simulink model "mixer_old"  (R2024b)
settings: Solver=FixedStepAuto  StartTime=0.0  StopTime=10.0  RelTol=1e-3
undefined symbols (not defined in the file or in its folder): MC_AIRMODE, MOT_SLEW_MAX, THR_MDL_FAC
libraries: simulink x58
(part 1 of 3)
settings Model: DataDictionary=nextpilot_datadict.sldd  Creator=DELL  LastModifiedBy=CETCA
settings DebuggingCC: UnconnectedInputMsg=warning  UnconnectedOutputMsg=warning  UnconnectedLineMsg=warning
settings ModelReferenceCC: EnableRefExpFcnMdlSchedulingChecks=on
settings RTWCC: GPUComputeCapability=3.5  DLArmComputeVersion=19.05

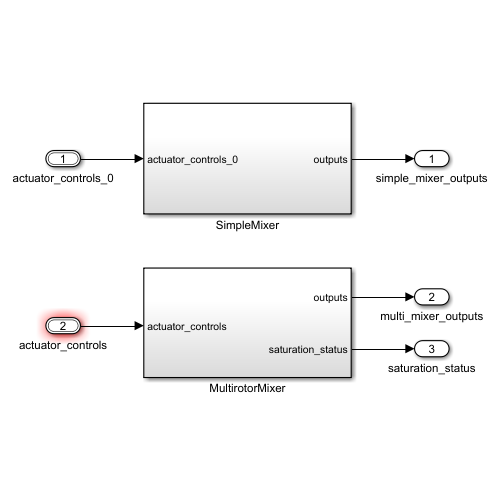
[thumbnail: Simulink's stored preview of the top-level diagram]
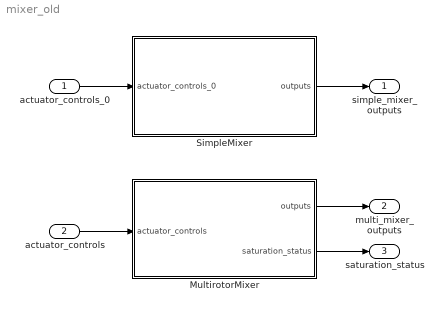
== system mixer_old ==
  actuator_controls_0 : Inport  OutDataTypeStr=Bus: actuator_controls_s
  actuator_controls : Inport  Port=2  OutDataTypeStr=Bus: px4_actuator_controls
  MultirotorMixer : Subsystem
  SimpleMixer : Subsystem
  simple_mixer_outputs : Outport
  multi_mixer_outputs : Outport  Port=2
  saturation_status : Outport  Port=3
  wires:
  actuator_controls/1 -> MultirotorMixer/1(actuator_controls)
  SimpleMixer/1(outputs) -> simple_mixer_outputs/1
  MultirotorMixer/1(outputs) -> multi_mixer_outputs/1
  MultirotorMixer/2(saturation_status) -> saturation_status/1
  actuator_controls_0/1 -> SimpleMixer/1(actuator_controls_0)

== system mixer_old/MultirotorMixer ==
  Bus Element In : Inport  PortName=actuator_controls  Element=control
  Bus Selector : BusSelector  OutputSignals=motor_neg,motor_pos,outputs
  Constant : Constant  Value=MC_AIRMODE
  Merge : Merge  Inputs=3
  Mux : Mux  Inputs=2
  Saturation : Saturate  UpperLimit=1.0  LowerLimit=-1.0
      settings: AttributesFormatString=[%<LowerLimit>, %<UpperLimit>]
  Saturation1 : Saturate  UpperLimit=1.0  LowerLimit=0.0
      settings: AttributesFormatString=[%<LowerLimit>, %<UpperLimit>]
  Selector : Selector  InputPortWidth=8  IndexOptions=Index vector (dialog)  Indices=[1 2 3]  OutputSizes=1
  Selector1 : Selector  InputPortWidth=8  IndexOptions=Index vector (dialog)  Indices=4  OutputSizes=1
  Switch Case : SwitchCase  CaseConditions={1 2}
  apply_thrust_model : Subsystem
  config_quad_x : Constant  Value=[-0.707107, 0.707107, 1.000000, 1.000000; 0.707107, -0.707107, 1.000000, 1.000000; 0.707107, 0.707107, -1.000000, 1.000000; -0.707107, -0.707107, -1.000000, 1.000000]  OutDataTypeStr=single
  mix_airmode_disabled : Subsystem
  mix_airmode_rp : Subsystem
  mix_airmode_rpy : Subsystem
  update_saturation_status : Subsystem
  outputs : Outport
  saturation_status : Outport  Port=2
  wires:
  Bus Element In/1 -> Selector1/1, Selector/1
  Selector/1 -> Saturation/1
  Selector1/1 -> Saturation1/1
  Saturation/1 -> Mux/1  "roll pitch yaw"
  Saturation1/1 -> Mux/2  "thrust"
  mix_airmode_rp/1(out) -> Merge/1
  mix_airmode_disabled/1(out) -> Merge/3
  Constant/1 -> Switch Case/1
  Switch Case/1 -> mix_airmode_rp/Action
  Switch Case/2 -> mix_airmode_rpy/Action
  Switch Case/3 -> mix_airmode_disabled/Action
  Mux/1 -> [four_channel]
  Merge/1 -> Bus Selector/1
  Bus Selector/1 -> [motor_neg]  "<motor_neg>"
  Bus Selector/2 -> [motor_pos]  "<motor_pos>"
  Bus Selector/3 -> apply_thrust_model/1(input)  "<outputs>"
  [motor_neg] -> update_saturation_status/2(motor_neg)
  [motor_pos] -> update_saturation_status/3(motor_pos)
  apply_thrust_model/2(clipping) -> update_saturation_status/1(clipping)
  apply_thrust_model/1(outputs) -> outputs/1
  update_saturation_status/1(saturation_status) -> saturation_status/1
  config_quad_x/1 -> [scale]
  [four_channel] -> mix_airmode_rp/1(four_input)
  [scale] -> mix_airmode_rp/2(scale)
  [four_channel] -> mix_airmode_rpy/1(four_input1)
  [scale] -> mix_airmode_rpy/2(scale1)
  mix_airmode_rpy/1(out1) -> Merge/2
  [four_channel] -> mix_airmode_disabled/1(four_input)
  [scale] -> mix_airmode_disabled/2(scale)
  [scale] -> update_saturation_status/4(scales)

== system mixer_old/SimpleMixer ==
  Bus Element In{,1..4} (5 alike) : Inport  PortName=actuator_controls_0  Element=control
  Constant{,1..19} (20 alike) : Constant  Value=[1 1]  OutDataTypeStr=single
  Constant{20..24} (5 alike) : Constant  OutDataTypeStr=single
  Mux : Mux  Inputs=5
  Selector : Selector  InputPortWidth=8  IndexOptions=Index vector (dialog)  Indices=[1 7]  OutputSizes=1
  Selector1 : Selector  InputPortWidth=8  IndexOptions=Index vector (dialog)  Indices=[1 7]  OutputSizes=1
  Selector2 : Selector  InputPortWidth=8  IndexOptions=Index vector (dialog)  Indices=[3 2]  OutputSizes=1
  Selector3 : Selector  InputPortWidth=8  IndexOptions=Index vector (dialog)  Indices=[3 2]  OutputSizes=1
  Selector4 : Selector  InputPortWidth=8  IndexOptions=Index vector (dialog)  Indices=4  OutputSizes=1
  Sum of Elements{,1..3} (4 alike) : Sum  Inputs=+
  scale : Subsystem
  scale1 : Subsystem
  scale2 : Subsystem
  scale3 : Subsystem
  scale4 : Subsystem
  outputs : Outport
  wires:
  Sum of Elements/1 -> [aileron_left]
  Sum of Elements1/1 -> [aileron_right]
  Sum of Elements3/1 -> [v_right]
  Sum of Elements2/1 -> [v_left]
  scale4/1(output) -> [prop]
  Bus Element In/1 -> Selector/1
  Bus Element In1/1 -> Selector1/1
  Bus Element In2/1 -> Selector2/1
  Bus Element In3/1 -> Selector3/1
  Bus Element In4/1 -> Selector4/1
  Constant4/1 -> scale/6(max)
  Selector/1 -> scale/1(input)
  Constant/1 -> scale/2(negative_scale)
  Constant3/1 -> scale/5(min)
  Constant1/1 -> scale/3(positive_scale)
  Constant2/1 -> scale/4(offset)
  scale/1(output) -> Sum of Elements/1
  scale1/1(output) -> Sum of Elements1/1
  Selector1/1 -> scale1/1(input)
  Constant5/1 -> scale1/2(negative_scale)
  Constant6/1 -> scale1/3(positive_scale)
  Constant7/1 -> scale1/4(offset)
  Constant8/1 -> scale1/5(min)
  Constant9/1 -> scale1/6(max)
  scale2/1(output) -> Sum of Elements2/1
  Selector2/1 -> scale2/1(input)
  Selector3/1 -> scale3/1(input)
  scale3/1(output) -> Sum of Elements3/1
  Selector4/1 -> scale4/1(input)
  Constant20/1 -> scale4/2(negative_scale)
  Constant10/1 -> scale2/2(negative_scale)
  Constant11/1 -> scale2/3(positive_scale)
  Constant12/1 -> scale2/4(offset)
  Constant13/1 -> scale2/5(min)
  Constant14/1 -> scale2/6(max)
  Constant15/1 -> scale3/2(negative_scale)
  Constant16/1 -> scale3/3(positive_scale)
  Constant17/1 -> scale3/4(offset)
  Constant18/1 -> scale3/5(min)
  Constant19/1 -> scale3/6(max)
  Constant21/1 -> scale4/3(positive_scale)
  Constant22/1 -> scale4/4(offset)
  Constant23/1 -> scale4/5(min)
  Constant24/1 -> scale4/6(max)
  [v_left] -> Mux/3
  [aileron_right] -> Mux/2
  [v_right] -> Mux/4
  [aileron_left] -> Mux/1
  [prop] -> Mux/5
  Mux/1 -> outputs/1

== system mixer_old/MultirotorMixer/apply_thrust_model ==
  input : Inport
  slew_rate_limit : Subsystem
  thrust_model : Subsystem
  outputs : Outport
  clipping : Outport  Port=2
  wires:
  input/1 -> thrust_model/1(input)
  thrust_model/1(outputs) -> slew_rate_limit/1(input)
  slew_rate_limit/2(clipping) -> clipping/1
  slew_rate_limit/1(output1) -> outputs/1

== system mixer_old/MultirotorMixer/mix_airmode_disabled ==
  four_input : Inport
  scale : Inport  Port=2
  Action Port : ActionPort  ActionPortLabel=default:
  Bus Selector3 : BusSelector  OutputSignals=outputs
  Bus Selector4 : BusSelector  OutputSignals=outputs
  Constant10 : Constant  OutDataTypeStr=single
  Constant11 : Constant  OutDataTypeStr=single
  Constant12 : Constant  Value=0  OutDataTypeStr=single
  Constant13 : Constant  OutDataTypeStr=single
  Constant14 : Constant  Value=0  OutDataTypeStr=single
  Constant9 : Constant  Value=0  OutDataTypeStr=single
  four_input1 : InportShadow
  minimize_saturation : Subsystem
  minimize_saturation1 : Subsystem
  minimize_saturation2 : Subsystem
  mix_yaw : Subsystem
  reduce_only : Constant  Value=0  OutDataTypeStr=single
  reduce_only1 : Constant  Value=0  OutDataTypeStr=single
  reduce_only2 : Constant  Value=0  OutDataTypeStr=single
  scale1 : InportShadow  Port=2
  scale2 : InportShadow  Port=2
  scale3 : InportShadow  Port=2
  out : Outport
  wires:
  scale/1 -> minimize_saturation/2(scale)
  reduce_only/1 -> minimize_saturation/5(reduce_only)
  Constant9/1 -> minimize_saturation/3(min_out)
  four_input/1 -> minimize_saturation/1(inputs)
  Constant10/1 -> minimize_saturation/4(max_out)
  Constant11/1 -> minimize_saturation1/4(max_out)
  Bus Selector3/1 -> minimize_saturation1/1(inputs)  "<outputs>"
  Constant12/1 -> minimize_saturation1/3(min_out)
  reduce_only1/1 -> minimize_saturation1/5(reduce_only)
  scale1/1 -> minimize_saturation1/2(scale)
  scale2/1 -> minimize_saturation2/2(scale)
  reduce_only2/1 -> minimize_saturation2/5(reduce_only)
  Constant14/1 -> minimize_saturation2/3(min_out)
  Bus Selector4/1 -> minimize_saturation2/1(inputs)  "<outputs>"
  Constant13/1 -> minimize_saturation2/4(max_out)
  minimize_saturation/1(out) -> Bus Selector3/1
  minimize_saturation1/1(out) -> Bus Selector4/1
  minimize_saturation2/1(out) -> mix_yaw/1(inputs)
  four_input1/1 -> mix_yaw/2(four_input)
  scale3/1 -> mix_yaw/3(scale)
  mix_yaw/1(out) -> out/1

== system mixer_old/MultirotorMixer/mix_airmode_rp ==
  four_input : Inport
  scale : Inport  Port=2
  Action Port : ActionPort  ActionPortLabel=case [ 1 ]:
  Constant1 : Constant  Value=0  OutDataTypeStr=single
  Constant2 : Constant  OutDataTypeStr=single
  four_input1 : InportShadow
  minimize_saturation : Subsystem
  mix_without_yaw : Subsystem
  mix_yaw : Subsystem
  reduce_only : Constant  Value=0  OutDataTypeStr=single
  scale1 : InportShadow  Port=2
  scale2 : InportShadow  Port=2
  out : Outport
  wires:
  reduce_only/1 -> minimize_saturation/5(reduce_only)
  four_input1/1 -> mix_yaw/2(four_input)
  Constant1/1 -> minimize_saturation/3(min_out)
  Constant2/1 -> minimize_saturation/4(max_out)
  minimize_saturation/1(out) -> mix_yaw/1(inputs)
  mix_yaw/1(out) -> out/1
  four_input/1 -> mix_without_yaw/1(four_input)
  scale/1 -> mix_without_yaw/2(scale)
  scale1/1 -> minimize_saturation/2(scale)
  mix_without_yaw/1(outputs) -> minimize_saturation/1(inputs)
  scale2/1 -> mix_yaw/3(scale)

== system mixer_old/MultirotorMixer/mix_airmode_rpy ==
  four_input1 : Inport
  scale1 : Inport  Port=2
  Action Port : ActionPort  ActionPortLabel=case [ 2 ]:
  Bus Selector : BusSelector  OutputSignals=outputs
  Constant6 : Constant  Value=0  OutDataTypeStr=single
  Constant7 : Constant  OutDataTypeStr=single
  Constant8 : Constant  Value=0  OutDataTypeStr=single
  Constant9 : Constant  OutDataTypeStr=single
  full_mixing : Subsystem
  minimize_saturation : Subsystem
  minimize_saturation1 : Subsystem
  reduce_only : Constant  Value=0  OutDataTypeStr=single
  reduce_only1 : Constant  Value=0  OutDataTypeStr=single
  scale2 : InportShadow  Port=2
  scale3 : InportShadow  Port=2
  out1 : Outport
  wires:
  four_input1/1 -> full_mixing/1(four_input)
  scale1/1 -> full_mixing/2(scale)
  scale2/1 -> minimize_saturation/2(scale)
  reduce_only/1 -> minimize_saturation/5(reduce_only)
  Constant6/1 -> minimize_saturation/3(min_out)
  full_mixing/1(outputs) -> minimize_saturation/1(inputs)
  Constant7/1 -> minimize_saturation/4(max_out)
  scale3/1 -> minimize_saturation1/2(scale)
  Constant8/1 -> minimize_saturation1/3(min_out)
  Constant9/1 -> minimize_saturation1/4(max_out)
  reduce_only1/1 -> minimize_saturation1/5(reduce_only)
  minimize_saturation1/1(out) -> out1/1
  minimize_saturation/1(out) -> Bus Selector/1
  Bus Selector/1 -> minimize_saturation1/1(inputs)  "<outputs>"

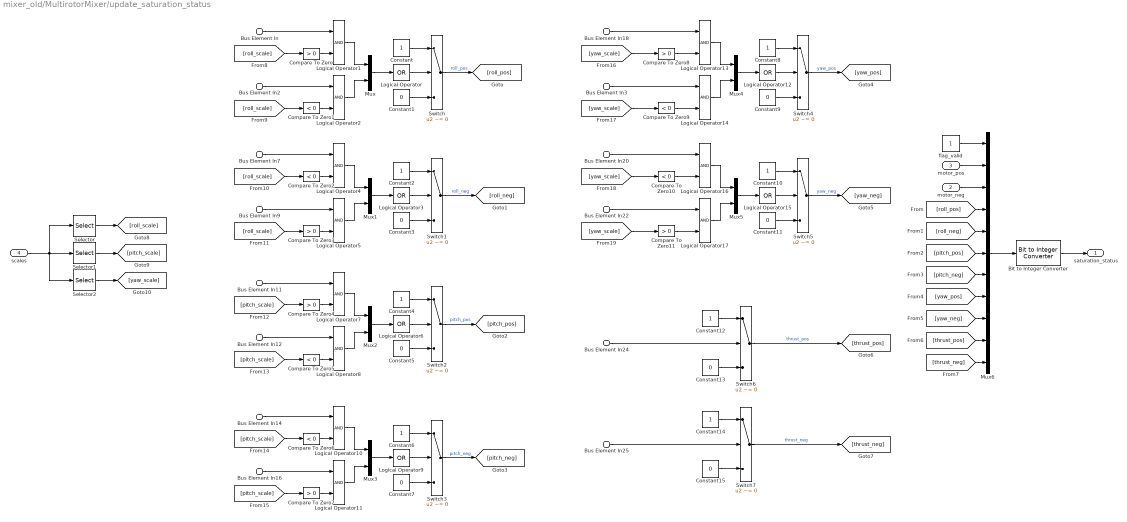
== system mixer_old/MultirotorMixer/update_saturation_status ==
  Bus Element In{,7,11,14,18,20,24} (7 alike) : Inport  PortName=clipping  Element=clipping_high
  Bus Element In{2,9,12,16,25} (5 alike) : Inport  PortName=clipping  Element=clipping_low_roll_pitch
  Bus Element In3 : Inport  PortName=clipping  Element=clipping_low_yaw
  Bus Element In22 : Inport  PortName=clipping  Element=clipping_low_yaw
  motor_neg : Inport  Port=2
  motor_pos : Inport  Port=3
  scales : Inport  Port=4
  Bit to Integer Converter : simulink/Logic and Bit Operations/Bit to Integer Converter  nbits=11  bitOrder=MSB first  signedOutputValues=Unsigned  outDtype=Inherit via internal rule  outDtypeSigned=Inherit via internal rule
      settings: LibrarySourceBlock=|
      | commutil2/Bit to Integer
      | Converter
  Compare To Zero{,3..4,7..8,11} (6 alike) : simulink/Logic and Bit Operations/Compare To Zero  relop=>  OutDataTypeStr=boolean
  Compare To Zero{1..2,5..6,9..10} (6 alike) : simulink/Logic and Bit Operations/Compare To Zero  relop=<  OutDataTypeStr=boolean
  Constant{,2,4,6,8,10,12,14} (8 alike) : Constant  OutDataTypeStr=single
  Constant{1,3,5,7,9,11,13,15} (8 alike) : Constant  Value=0  OutDataTypeStr=single
  Logical Operator{,3,6,9,12,15} (6 alike) : Logic  Operator=OR  Inputs=1  AllPortsSameDT=off  OutDataTypeStr=boolean
  Logical Operator{1..2,4..5,7..8,10..11,13..14,16..17} (12 alike) : Logic  AllPortsSameDT=off  OutDataTypeStr=boolean
  Mux{,1..5} (6 alike) : Mux  Inputs=2
  Mux6 : Mux  Inputs=11
  Selector : Selector  NumberOfDimensions=2  InputPortWidth=3  IndexOptions=Select all,Index vector (dialog)  Indices=[1 3],1  OutputSizes=1,1
  Selector1 : Selector  NumberOfDimensions=2  InputPortWidth=3  IndexOptions=Select all,Index vector (dialog)  Indices=[1 3],2  OutputSizes=1,1
  Selector2 : Selector  NumberOfDimensions=2  InputPortWidth=3  IndexOptions=Select all,Index vector (dialog)  Indices=[1 3],3  OutputSizes=1,1
  Switch{,1..7} (8 alike) : Switch  Criteria=u2 ~= 0  SaturateOnIntegerOverflow=off  InputSameDT=off
  flag_valid : Constant  OutDataTypeStr=single
  saturation_status : Outport
  wires:
  Switch/1 -> [roll_pos]  "roll_pos"
  Constant/1 -> Switch/1
  Constant1/1 -> Switch/3
  Logical Operator/1 -> Switch/2
  Bus Element In/1 -> Logical Operator1/1
  Compare To Zero/1 -> Logical Operator1/2
  [roll_scale] -> Compare To Zero/1
  Bus Element In2/1 -> Logical Operator2/1
  Compare To Zero1/1 -> Logical Operator2/2
  [roll_scale] -> Compare To Zero1/1
  Mux/1 -> Logical Operator/1
  Logical Operator1/1 -> Mux/1
  Logical Operator2/1 -> Mux/2
  Switch1/1 -> [roll_neg]  "roll_neg"
  Constant2/1 -> Switch1/1
  Constant3/1 -> Switch1/3
  Mux1/1 -> Logical Operator3/1
  Logical Operator3/1 -> Switch1/2
  Logical Operator4/1 -> Mux1/1
  Logical Operator5/1 -> Mux1/2
  Bus Element In7/1 -> Logical Operator4/1
  [roll_scale] -> Compare To Zero2/1
  Compare To Zero2/1 -> Logical Operator4/2
  Bus Element In9/1 -> Logical Operator5/1
  [roll_scale] -> Compare To Zero3/1
  Compare To Zero3/1 -> Logical Operator5/2
  Logical Operator6/1 -> Switch2/2
  Constant5/1 -> Switch2/3
  Constant4/1 -> Switch2/1
  Switch2/1 -> [pitch_pos]  "pitch_pos"
  Logical Operator8/1 -> Mux2/2
  Logical Operator7/1 -> Mux2/1
  Mux2/1 -> Logical Operator6/1
  Bus Element In11/1 -> Logical Operator7/1
  [pitch_scale] -> Compare To Zero4/1
  Compare To Zero4/1 -> Logical Operator7/2
  Bus Element In12/1 -> Logical Operator8/1
  Compare To Zero5/1 -> Logical Operator8/2
  [pitch_scale] -> Compare To Zero5/1
  Mux3/1 -> Logical Operator9/1
  Logical Operator10/1 -> Mux3/1
  Logical Operator11/1 -> Mux3/2
  Switch3/1 -> [pitch_neg]  "pitch_neg"
  Constant6/1 -> Switch3/1
  Constant7/1 -> Switch3/3
  Logical Operator9/1 -> Switch3/2
  Bus Element In14/1 -> Logical Operator10/1
  [pitch_scale] -> Compare To Zero6/1
  Compare To Zero6/1 -> Logical Operator10/2
  Bus Element In16/1 -> Logical Operator11/1
  [pitch_scale] -> Compare To Zero7/1
  Compare To Zero7/1 -> Logical Operator11/2
  Logical Operator14/1 -> Mux4/2
  Logical Operator13/1 -> Mux4/1
  Mux4/1 -> Logical Operator12/1
  Logical Operator12/1 -> Switch4/2
  Constant9/1 -> Switch4/3
  Constant8/1 -> Switch4/1
  Switch4/1 -> [yaw_pos]  "yaw_pos"
  Bus Element In18/1 -> Logical Operator13/1
  Compare To Zero8/1 -> Logical Operator13/2
  [yaw_scale] -> Compare To Zero8/1
  Bus Element In3/1 -> Logical Operator14/1
  Compare To Zero9/1 -> Logical Operator14/2
  [yaw_scale] -> Compare To Zero9/1
  Switch5/1 -> [yaw_neg]  "yaw_neg"
  Constant10/1 -> Switch5/1
  Constant11/1 -> Switch5/3
  Logical Operator15/1 -> Switch5/2
  Mux5/1 -> Logical Operator15/1
  Logical Operator16/1 -> Mux5/1
  Logical Operator17/1 -> Mux5/2
  Bus Element In20/1 -> Logical Operator16/1
  [yaw_scale] -> Compare To Zero10/1
  Compare To Zero10/1 -> Logical Operator16/2
  Bus Element In22/1 -> Logical Operator17/1
  [yaw_scale] -> Compare To Zero11/1
  Compare To Zero11/1 -> Logical Operator17/2
  Bus Element In24/1 -> Switch6/2
  Constant13/1 -> Switch6/3
  Constant12/1 -> Switch6/1
  Switch6/1 -> [thrust_pos]  "thrust_pos"
  Switch7/1 -> [thrust_neg]  "thrust_neg"
  Constant14/1 -> Switch7/1
  Constant15/1 -> Switch7/3
  Bus Element In25/1 -> Switch7/2
  Bit to Integer Converter/1 -> saturation_status/1
  Mux6/1 -> Bit to Integer Converter/1
  flag_valid/1 -> Mux6/1
  motor_pos/1 -> Mux6/2
  motor_neg/1 -> Mux6/3
  [roll_pos] -> Mux6/4
  [roll_neg] -> Mux6/5
  [pitch_pos] -> Mux6/6
  [pitch_neg] -> Mux6/7
  [yaw_pos] -> Mux6/8
  [yaw_neg] -> Mux6/9
  [thrust_pos] -> Mux6/10
  [thrust_neg] -> Mux6/11
  scales/1 -> Selector/1, Selector2/1, Selector1/1
  Selector/1 -> [roll_scale]
  Selector1/1 -> [pitch_scale]
  Selector2/1 -> [yaw_scale]

== system mixer_old/SimpleMixer/scale ==
  input : Inport
  negative_scale : Inport  Port=2
  positive_scale : Inport  Port=3
  offset : Inport  Port=4
  min : Inport  Port=5
  max : Inport  Port=6
  Product : Product
  Saturation Dynamic : simulink/Discontinuities/Saturation Dynamic  OutMin=[]  OutMax=[]  OutDataTypeStr=Inherit: Same as second input  OutDataType=fixdt(1, 16)  OutScaling=2^-10  DoSatur=off
  Sum : Sum  Inputs=|++
  Switch : Switch  SaturateOnIntegerOverflow=off  InputSameDT=off
  input1 : InportShadow
  output : Outport
  wires:
  input/1 -> Switch/2
  positive_scale/1 -> Switch/1
  negative_scale/1 -> Switch/3
  Switch/1 -> Product/2
  input1/1 -> Product/1
  Product/1 -> Sum/1
  offset/1 -> Sum/2
  max/1 -> Saturation Dynamic/1
  min/1 -> Saturation Dynamic/3
  Sum/1 -> Saturation Dynamic/2
  Saturation Dynamic/1 -> output/1

== system mixer_old/SimpleMixer/scale1 ==
  input : Inport
  negative_scale : Inport  Port=2
  positive_scale : Inport  Port=3
  offset : Inport  Port=4
  min : Inport  Port=5
  max : Inport  Port=6
  Product : Product
  Saturation Dynamic : simulink/Discontinuities/Saturation Dynamic  OutMin=[]  OutMax=[]  OutDataTypeStr=Inherit: Same as second input  OutDataType=fixdt(1, 16)  OutScaling=2^-10  DoSatur=off
  Sum : Sum  Inputs=|++
  Switch : Switch  SaturateOnIntegerOverflow=off  InputSameDT=off
  input1 : InportShadow
  output : Outport
  wires:
  Saturation Dynamic/1 -> output/1
  Sum/1 -> Saturation Dynamic/2
  min/1 -> Saturation Dynamic/3
  max/1 -> Saturation Dynamic/1
  offset/1 -> Sum/2
  Product/1 -> Sum/1
  input1/1 -> Product/1
  Switch/1 -> Product/2
  negative_scale/1 -> Switch/3
  positive_scale/1 -> Switch/1
  input/1 -> Switch/2

== system mixer_old/SimpleMixer/scale2 ==
  input : Inport
  negative_scale : Inport  Port=2
  positive_scale : Inport  Port=3
  offset : Inport  Port=4
  min : Inport  Port=5
  max : Inport  Port=6
  Product : Product
  Saturation Dynamic : simulink/Discontinuities/Saturation Dynamic  OutMin=[]  OutMax=[]  OutDataTypeStr=Inherit: Same as second input  OutDataType=fixdt(1, 16)  OutScaling=2^-10  DoSatur=off
  Sum : Sum  Inputs=|++
  Switch : Switch  SaturateOnIntegerOverflow=off  InputSameDT=off
  input1 : InportShadow
  output : Outport
  wires:
  Saturation Dynamic/1 -> output/1
  Sum/1 -> Saturation Dynamic/2
  min/1 -> Saturation Dynamic/3
  max/1 -> Saturation Dynamic/1
  offset/1 -> Sum/2
  Product/1 -> Sum/1
  input1/1 -> Product/1
  Switch/1 -> Product/2
  negative_scale/1 -> Switch/3
  positive_scale/1 -> Switch/1
  input/1 -> Switch/2

== system mixer_old/SimpleMixer/scale3 ==
  input : Inport
  negative_scale : Inport  Port=2
  positive_scale : Inport  Port=3
  offset : Inport  Port=4
  min : Inport  Port=5
  max : Inport  Port=6
  Product : Product
  Saturation Dynamic : simulink/Discontinuities/Saturation Dynamic  OutMin=[]  OutMax=[]  OutDataTypeStr=Inherit: Same as second input  OutDataType=fixdt(1, 16)  OutScaling=2^-10  DoSatur=off
  Sum : Sum  Inputs=|++
  Switch : Switch  SaturateOnIntegerOverflow=off  InputSameDT=off
  input1 : InportShadow
  output : Outport
  wires:
  input/1 -> Switch/2
  positive_scale/1 -> Switch/1
  negative_scale/1 -> Switch/3
  Switch/1 -> Product/2
  input1/1 -> Product/1
  Product/1 -> Sum/1
  offset/1 -> Sum/2
  max/1 -> Saturation Dynamic/1
  min/1 -> Saturation Dynamic/3
  Sum/1 -> Saturation Dynamic/2
  Saturation Dynamic/1 -> output/1

== system mixer_old/SimpleMixer/scale4 ==
  input : Inport
  negative_scale : Inport  Port=2
  positive_scale : Inport  Port=3
  offset : Inport  Port=4
  min : Inport  Port=5
  max : Inport  Port=6
  Product : Product
  Saturation Dynamic : simulink/Discontinuities/Saturation Dynamic  OutMin=[]  OutMax=[]  OutDataTypeStr=Inherit: Same as second input  OutDataType=fixdt(1, 16)  OutScaling=2^-10  DoSatur=off
  Sum : Sum  Inputs=|++
  Switch : Switch  SaturateOnIntegerOverflow=off  InputSameDT=off
  input1 : InportShadow
  output : Outport
  wires:
  input/1 -> Switch/2
  positive_scale/1 -> Switch/1
  negative_scale/1 -> Switch/3
  Switch/1 -> Product/2
  input1/1 -> Product/1
  Product/1 -> Sum/1
  offset/1 -> Sum/2
  max/1 -> Saturation Dynamic/1
  min/1 -> Saturation Dynamic/3
  Sum/1 -> Saturation Dynamic/2
  Saturation Dynamic/1 -> output/1

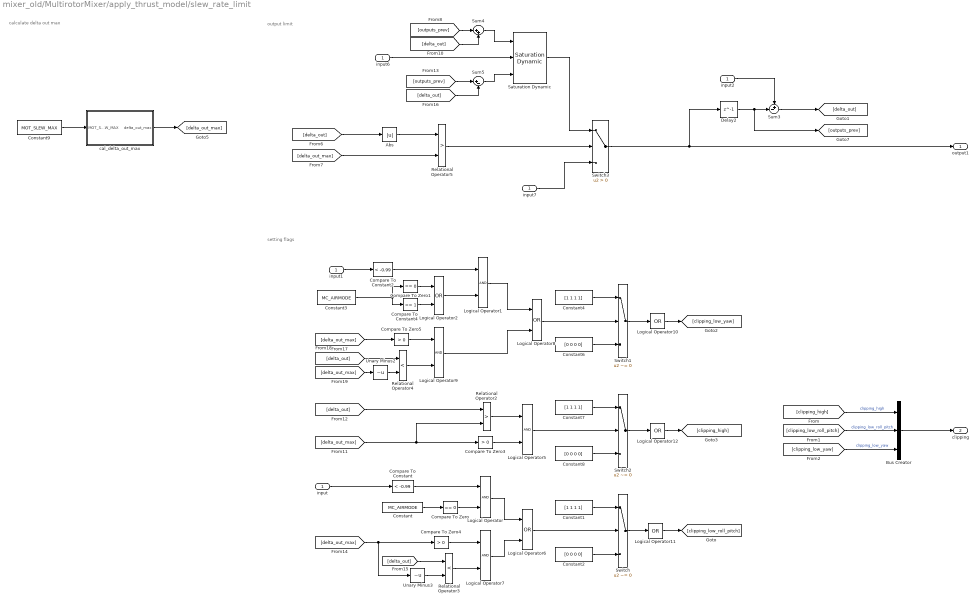
== system mixer_old/MultirotorMixer/apply_thrust_model/slew_rate_limit ==
  note: output limit
  note: setting flags
  note: calculate delta out max
  input : Inport
  Abs : Abs  SaturateOnIntegerOverflow=off
  Bus Creator : BusCreator  Inputs=3
  Compare To Constant : simulink/Logic and Bit Operations/Compare To Constant  relop=<  const=-0.99  OutDataTypeStr=boolean
  Compare To Constant2 : simulink/Logic and Bit Operations/Compare To Constant  relop=<  const=-0.99  OutDataTypeStr=boolean
  Compare To Constant4 : simulink/Logic and Bit Operations/Compare To Constant  relop===  const=1  OutDataTypeStr=boolean
  Compare To Zero : simulink/Logic and Bit Operations/Compare To Zero  relop===  OutDataTypeStr=boolean
  Compare To Zero1 : simulink/Logic and Bit Operations/Compare To Zero  relop===  OutDataTypeStr=boolean
  Compare To Zero3 : simulink/Logic and Bit Operations/Compare To Zero  relop=>  OutDataTypeStr=boolean
  Compare To Zero4 : simulink/Logic and Bit Operations/Compare To Zero  relop=>  OutDataTypeStr=boolean
  Compare To Zero5 : simulink/Logic and Bit Operations/Compare To Zero  relop=>  OutDataTypeStr=boolean
  Constant : Constant  Value=MC_AIRMODE
  Constant1 : Constant  Value=[1 1 1 1]  OutDataTypeStr=boolean
  Constant2 : Constant  Value=[0 0 0 0]  OutDataTypeStr=boolean
  Constant3 : Constant  Value=MC_AIRMODE
  Constant4 : Constant  Value=[1 1 1 1]  OutDataTypeStr=boolean
  Constant6 : Constant  Value=[0 0 0 0]  OutDataTypeStr=boolean
  Constant7 : Constant  Value=[1 1 1 1]  OutDataTypeStr=boolean
  Constant8 : Constant  Value=[0 0 0 0]  OutDataTypeStr=boolean
  Constant9 : Constant  Value=MOT_SLEW_MAX
  Delay2 : Delay  DelayLength=1
  Logical Operator{,1,5,7,9} (5 alike) : Logic  AllPortsSameDT=off  OutDataTypeStr=boolean
  Logical Operator10 : Logic  Operator=OR  Inputs=1  AllPortsSameDT=off  OutDataTypeStr=boolean
  Logical Operator11 : Logic  Operator=OR  Inputs=1  AllPortsSameDT=off  OutDataTypeStr=boolean
  Logical Operator12 : Logic  Operator=OR  Inputs=1  AllPortsSameDT=off  OutDataTypeStr=boolean
  Logical Operator2 : Logic  Operator=OR  AllPortsSameDT=off  OutDataTypeStr=boolean
  Logical Operator6 : Logic  Operator=OR  AllPortsSameDT=off  OutDataTypeStr=boolean
  Logical Operator8 : Logic  Operator=OR  AllPortsSameDT=off  OutDataTypeStr=boolean
  Relational Operator2 : RelationalOperator  Operator=>  OutDataTypeStr=boolean  RndMeth=Simplest  InputSameDT=off
  Relational Operator3 : RelationalOperator  Operator=<  OutDataTypeStr=boolean  RndMeth=Simplest  InputSameDT=off
  Relational Operator4 : RelationalOperator  Operator=<  OutDataTypeStr=boolean  RndMeth=Simplest  InputSameDT=off
  Relational Operator5 : RelationalOperator  Operator=>  OutDataTypeStr=boolean  RndMeth=Simplest  InputSameDT=off
  Saturation Dynamic : simulink/Discontinuities/Saturation Dynamic  OutMin=[]  OutMax=[]  OutDataTypeStr=Inherit: Same as second input  OutDataType=fixdt(1, 16)  OutScaling=2^-10  DoSatur=off
  Sum3 : Sum  Inputs=+-|
  Sum4 : Sum  Inputs=|++
  Sum5 : Sum  Inputs=|+-
  Switch : Switch  Criteria=u2 ~= 0  SaturateOnIntegerOverflow=off  InputSameDT=off
  Switch1 : Switch  Criteria=u2 ~= 0  SaturateOnIntegerOverflow=off  InputSameDT=off
  Switch2 : Switch  Criteria=u2 ~= 0  SaturateOnIntegerOverflow=off  InputSameDT=off
  Switch3 : Switch  Criteria=u2 > Threshold  SaturateOnIntegerOverflow=off  InputSameDT=off
  Unary Minus2 : UnaryMinus
  Unary Minus3 : UnaryMinus
  cal_delta_out_max : Subsystem
  input{1..2,6..7} (4 alike) : InportShadow
  output1 : Outport
  clipping : Outport  Port=2
  wires:
  input/1 -> Compare To Constant/1
  Compare To Constant/1 -> Logical Operator/1
  Constant/1 -> Compare To Zero/1
  Compare To Zero/1 -> Logical Operator/2
  Constant1/1 -> Switch/1
  Constant2/1 -> Switch/3
  Compare To Constant2/1 -> Logical Operator1/1
  input1/1 -> Compare To Constant2/1
  Logical Operator2/1 -> Logical Operator1/2
  Compare To Zero1/1 -> Logical Operator2/1
  Constant3/1 -> Compare To Zero1/1, Compare To Constant4/1
  Compare To Constant4/1 -> Logical Operator2/2
  Constant6/1 -> Switch1/3
  Constant4/1 -> Switch1/1
  Switch2/1 -> Logical Operator12/1
  Bus Creator/1 -> clipping/1
  [clipping_high] -> Bus Creator/1  "clipping_high"
  [clipping_low_roll_pitch] -> Bus Creator/2  "clipping_low_roll_pitch"
  [clipping_low_yaw] -> Bus Creator/3  "clipping_low_yaw"
  Constant7/1 -> Switch2/1
  Constant8/1 -> Switch2/3
  Logical Operator5/1 -> Switch2/2
  [delta_out_max] -> Relational Operator2/2, Compare To Zero3/1
  [delta_out] -> Relational Operator2/1
  Logical Operator/1 -> Logical Operator6/1
  Logical Operator6/1 -> Switch/2
  Compare To Zero4/1 -> Logical Operator7/1
  [delta_out_max] -> Unary Minus3/1, Compare To Zero4/1
  Unary Minus3/1 -> Relational Operator3/2
  [delta_out] -> Relational Operator3/1
  Relational Operator3/1 -> Logical Operator7/2
  Logical Operator7/1 -> Logical Operator6/2
  Logical Operator8/1 -> Switch1/2
  Logical Operator1/1 -> Logical Operator8/1
  Relational Operator4/1 -> Logical Operator9/2
  [delta_out] -> Relational Operator4/1
  Unary Minus2/1 -> Relational Operator4/2
  [delta_out_max] -> Unary Minus2/1
  Compare To Zero5/1 -> Logical Operator9/1
  [delta_out_max] -> Compare To Zero5/1
  Logical Operator9/1 -> Logical Operator8/2
  Constant9/1 -> cal_delta_out_max/1(MOT_SLEW_MAX)
  cal_delta_out_max/1(delta_out_max) -> [delta_out_max]
  Switch1/1 -> Logical Operator10/1
  Logical Operator10/1 -> [clipping_low_yaw]
  Logical Operator12/1 -> [clipping_high]
  Switch/1 -> Logical Operator11/1
  Logical Operator11/1 -> [clipping_low_roll_pitch]
  [delta_out] -> Abs/1
  [delta_out_max] -> Relational Operator5/2
  Abs/1 -> Relational Operator5/1
  Relational Operator5/1 -> Switch3/2
  Delay2/1 -> [outputs_prev], Sum3/2
  Sum3/1 -> [delta_out]
  input2/1 -> Sum3/1
  Switch3/1 -> Delay2/1, output1/1
  Saturation Dynamic/1 -> Switch3/1
  input6/1 -> Saturation Dynamic/2
  input7/1 -> Switch3/3
  [outputs_prev] -> Sum4/1
  [delta_out] -> Sum4/2
  Sum4/1 -> Saturation Dynamic/1
  Sum5/1 -> Saturation Dynamic/3
  [outputs_prev] -> Sum5/1
  [delta_out] -> Sum5/2
  Compare To Zero3/1 -> Logical Operator5/2
  Relational Operator2/1 -> Logical Operator5/1

== system mixer_old/MultirotorMixer/apply_thrust_model/thrust_model ==
  note: $thrust = (1 - \_thrust\_factor) \times PWM + \_thrust\_factor \times PWM^2$
  input : Inport
  Constant : Constant  OutDataTypeStr=single
  Constant1 : Constant  Value=[1 1 1 1]  OutDataTypeStr=single
  Constant2 : Constant  Value=THR_MDL_FAC
      settings: AttributesFormatString=%<Value>
  Constant3 : Constant  Value=[0 0 0 0]  OutDataTypeStr=single
  Constant5 : Constant
  Divide : Product  Inputs=*/
  Divide1 : Product  Inputs=/*
  Divide2 : Product  Inputs=*/
  Gain : Gain  Gain=2
  Gain1 : Gain  Gain=2
  Gain2 : Gain  Gain=4
  Math Function1 : Math  Operator=square
  Math Function2 : Math  Operator=square
  Saturation : Saturate  UpperLimit=1  LowerLimit=-1
      settings: AttributesFormatString=[%<LowerLimit>, %<UpperLimit>]
  Saturation1 : Saturate  UpperLimit=1  LowerLimit=0
      settings: AttributesFormatString=[%<LowerLimit>, %<UpperLimit>]
  Sqrt : Sqrt
  Sum : Sum  Inputs=|+-
  Sum2 : Sum  Inputs=|+-
  Sum3 : Sum
  Sum4 : Sum  Inputs=|+-
  Sum5 : Sum  Inputs=++|
  Switch : Switch  Criteria=u2 > Threshold  SaturateOnIntegerOverflow=off  InputSameDT=off
  Switch1 : Switch  SaturateOnIntegerOverflow=off  InputSameDT=off
  input1 : InportShadow
  outputs : Outport
  wires:
  Constant2/1 -> Saturation1/1
  Saturation1/1 -> Sum4/1, Gain/1, [thrust_factor]
  Gain/1 -> Divide/2
  input1/1 -> Divide1/2, Switch1/2
  Constant3/1 -> Switch1/3
  Switch/1 -> Gain1/1  "outputs"
  input/1 -> Switch/3
  Gain1/1 -> Sum/1
  Divide/1 -> Sum5/2
  Saturation/1 -> outputs/1
  Sum5/1 -> Switch/1
  Divide1/1 -> Switch1/1
  Sum3/1 -> Sqrt/1
  Constant1/1 -> Sum/2
  Sum/1 -> Saturation/1
  [thrust_factor] -> Switch/2
  Sqrt/1 -> Sum5/1
  Constant5/1 -> Sum4/2
  Sum4/1 -> Divide/1
  Switch1/1 -> Sum3/2
  Constant/1 -> Sum2/1
  [thrust_factor] -> Divide1/1, Math Function2/1, Sum2/2
  Sum2/1 -> Math Function1/1
  Math Function1/1 -> Divide2/1
  Math Function2/1 -> Gain2/1
  Gain2/1 -> Divide2/2
  Divide2/1 -> Sum3/1

== system mixer_old/MultirotorMixer/mix_airmode_disabled/minimize_saturation ==
  inputs : Inport
  scale : Inport  Port=2
  min_out : Inport  Port=3
  max_out : Inport  Port=4
  reduce_only : Inport  Port=5
  Compare To Zero : simulink/Logic and Bit Operations/Compare To Zero  relop=>  OutDataTypeStr=boolean
  Data Type Conversion : DataTypeConversion  OutDataTypeStr=boolean  SaturateOnIntegerOverflow=off  RndMeth=Floor
  If : If  IfExpression=u1
  If Action Subsystem : Subsystem  TreatAsAtomicUnit=on
  Logical Operator : Logic  AllPortsSameDT=off  OutDataTypeStr=boolean
  Merge : Merge
  Subsystem : Subsystem
  compute_desaturation_gain : Subsystem
  inputs1 : InportShadow
  inputs2 : InportShadow
  scale1 : InportShadow  Port=2
  out : Outport
  wires:
  scale/1 -> compute_desaturation_gain/2(scale)
  inputs/1 -> compute_desaturation_gain/1(inputs)
  compute_desaturation_gain/3(k) -> [k1]
  reduce_only/1 -> Data Type Conversion/1
  [k1] -> Compare To Zero/1
  Data Type Conversion/1 -> Logical Operator/1
  Compare To Zero/1 -> Logical Operator/2
  Logical Operator/1 -> If/1
  Merge/1 -> out/1
  compute_desaturation_gain/2(motor_pos) -> [motor_pos]
  compute_desaturation_gain/1(motor_neg) -> [motor_neg]
  If/1 -> If Action Subsystem/Action
  scale1/1 -> Subsystem/2(scale)
  inputs2/1 -> Subsystem/3(inputs)
  If/2 -> Subsystem/Action
  [k1] -> Subsystem/1(k1)
  If Action Subsystem/1(out) -> Merge/1
  Subsystem/1(out) -> Merge/2
  [motor_pos] -> If Action Subsystem/2(motor_pos)
  [motor_neg] -> If Action Subsystem/1(motor_neg)
  inputs1/1 -> If Action Subsystem/3(outputs)
  min_out/1 -> compute_desaturation_gain/3(min)
  max_out/1 -> compute_desaturation_gain/4(max)

== system mixer_old/MultirotorMixer/mix_airmode_disabled/minimize_saturation1 ==
  inputs : Inport
  scale : Inport  Port=2
  min_out : Inport  Port=3
  max_out : Inport  Port=4
  reduce_only : Inport  Port=5
  Compare To Zero : simulink/Logic and Bit Operations/Compare To Zero  relop=>  OutDataTypeStr=boolean
  Data Type Conversion : DataTypeConversion  OutDataTypeStr=boolean  SaturateOnIntegerOverflow=off  RndMeth=Floor
  If : If  IfExpression=u1
  If Action Subsystem : Subsystem  TreatAsAtomicUnit=on
  Logical Operator : Logic  AllPortsSameDT=off  OutDataTypeStr=boolean
  Merge : Merge
  Subsystem : Subsystem
  compute_desaturation_gain : Subsystem
  inputs1 : InportShadow
  inputs2 : InportShadow
  scale1 : InportShadow  Port=2
  out : Outport
  wires:
  max_out/1 -> compute_desaturation_gain/4(max)
  min_out/1 -> compute_desaturation_gain/3(min)
  inputs1/1 -> If Action Subsystem/3(outputs)
  [motor_neg] -> If Action Subsystem/1(motor_neg)
  [motor_pos] -> If Action Subsystem/2(motor_pos)
  Subsystem/1(out) -> Merge/2
  If Action Subsystem/1(out) -> Merge/1
  [k1] -> Subsystem/1(k1)
  If/2 -> Subsystem/Action
  inputs2/1 -> Subsystem/3(inputs)
  scale1/1 -> Subsystem/2(scale)
  If/1 -> If Action Subsystem/Action
  compute_desaturation_gain/1(motor_neg) -> [motor_neg]
  compute_desaturation_gain/2(motor_pos) -> [motor_pos]
  Merge/1 -> out/1
  Logical Operator/1 -> If/1
  Compare To Zero/1 -> Logical Operator/2
  Data Type Conversion/1 -> Logical Operator/1
  [k1] -> Compare To Zero/1
  reduce_only/1 -> Data Type Conversion/1
  compute_desaturation_gain/3(k) -> [k1]
  inputs/1 -> compute_desaturation_gain/1(inputs)
  scale/1 -> compute_desaturation_gain/2(scale)

== system mixer_old/MultirotorMixer/mix_airmode_disabled/minimize_saturation2 ==
  inputs : Inport
  scale : Inport  Port=2
  min_out : Inport  Port=3
  max_out : Inport  Port=4
  reduce_only : Inport  Port=5
  Compare To Zero : simulink/Logic and Bit Operations/Compare To Zero  relop=>  OutDataTypeStr=boolean
  Data Type Conversion : DataTypeConversion  OutDataTypeStr=boolean  SaturateOnIntegerOverflow=off  RndMeth=Floor
  If : If  IfExpression=u1
  If Action Subsystem : Subsystem  TreatAsAtomicUnit=on
  Logical Operator : Logic  AllPortsSameDT=off  OutDataTypeStr=boolean
  Merge : Merge
  Subsystem : Subsystem
  compute_desaturation_gain : Subsystem
  inputs1 : InportShadow
  inputs2 : InportShadow
  scale1 : InportShadow  Port=2
  out : Outport
  wires:
  scale/1 -> compute_desaturation_gain/2(scale)
  inputs/1 -> compute_desaturation_gain/1(inputs)
  compute_desaturation_gain/3(k) -> [k1]
  reduce_only/1 -> Data Type Conversion/1
  [k1] -> Compare To Zero/1
  Data Type Conversion/1 -> Logical Operator/1
  Compare To Zero/1 -> Logical Operator/2
  Logical Operator/1 -> If/1
  Merge/1 -> out/1
  compute_desaturation_gain/2(motor_pos) -> [motor_pos]
  compute_desaturation_gain/1(motor_neg) -> [motor_neg]
  If/1 -> If Action Subsystem/Action
  scale1/1 -> Subsystem/2(scale)
  inputs2/1 -> Subsystem/3(inputs)
  If/2 -> Subsystem/Action
  [k1] -> Subsystem/1(k1)
  If Action Subsystem/1(out) -> Merge/1
  Subsystem/1(out) -> Merge/2
  [motor_pos] -> If Action Subsystem/2(motor_pos)
  [motor_neg] -> If Action Subsystem/1(motor_neg)
  inputs1/1 -> If Action Subsystem/3(outputs)
  min_out/1 -> compute_desaturation_gain/3(min)
  max_out/1 -> compute_desaturation_gain/4(max)

== system mixer_old/MultirotorMixer/mix_airmode_disabled/mix_yaw ==
  inputs : Inport
  four_input : Inport  Port=2
  scale : Inport  Port=3
  Bus Selector1 : BusSelector  OutputSignals=outputs
  Bus Selector2 : BusSelector  OutputSignals=outputs
  Constant : Constant  Value=0  OutDataTypeStr=single
  Constant1 : Constant  Value=1.15  OutDataTypeStr=single
  Constant2 : Constant  Value=0  OutDataTypeStr=single
  Constant3 : Constant  Value=0  OutDataTypeStr=single
  Constant4 : Constant  OutDataTypeStr=single
  Constant5 : Constant  OutDataTypeStr=single
  Product : Product
  Selector : Selector  InputPortWidth=4  IndexOptions=Index vector (dialog)  Indices=3  OutputSizes=1
  Selector1 : Selector  NumberOfDimensions=2  InputPortWidth=3  IndexOptions=Select all,Index vector (dialog)  Indices=[1 3],3  OutputSizes=1,1
  Sum : Sum  Inputs=++|
  minimize_saturation2 : Subsystem
  minimize_saturation3 : Subsystem
  scale1 : InportShadow  Port=3
  scale2 : InportShadow  Port=3
  out : Outport
  wires:
  four_input/1 -> Selector/1
  Selector/1 -> Product/1  "yaw"
  Product/1 -> Sum/2
  inputs/1 -> Bus Selector1/1
  scale/1 -> Selector1/1
  Selector1/1 -> Product/2  "yaw_scale"
  Bus Selector1/1 -> Sum/1  "<outputs>"
  Sum/1 -> minimize_saturation2/1(inputs)  "outputs"
  scale1/1 -> minimize_saturation2/2(scale)
  Constant2/1 -> minimize_saturation2/5(reduce_only)
  Constant1/1 -> minimize_saturation2/4(max_out)
  Constant/1 -> minimize_saturation2/3(min_out)
  minimize_saturation2/1(out) -> Bus Selector2/1
  Bus Selector2/1 -> minimize_saturation3/1(inputs)  "<outputs>"
  scale2/1 -> minimize_saturation3/2(scale)
  Constant5/1 -> minimize_saturation3/5(reduce_only)
  Constant3/1 -> minimize_saturation3/3(min_out)
  Constant4/1 -> minimize_saturation3/4(max_out)
  minimize_saturation3/1(out) -> out/1

== system mixer_old/MultirotorMixer/mix_airmode_rp/minimize_saturation ==
  inputs : Inport
  scale : Inport  Port=2
  min_out : Inport  Port=3
  max_out : Inport  Port=4
  reduce_only : Inport  Port=5
  Compare To Zero : simulink/Logic and Bit Operations/Compare To Zero  relop=>  OutDataTypeStr=boolean
  Data Type Conversion : DataTypeConversion  OutDataTypeStr=boolean  SaturateOnIntegerOverflow=off  RndMeth=Floor
  If : If  IfExpression=u1
  If Action Subsystem : Subsystem  TreatAsAtomicUnit=on
  Logical Operator : Logic  AllPortsSameDT=off  OutDataTypeStr=boolean
  Merge : Merge
  Subsystem : Subsystem
  compute_desaturation_gain : Subsystem
  inputs1 : InportShadow
  inputs2 : InportShadow
  scale1 : InportShadow  Port=2
  out : Outport
  wires:
  scale/1 -> compute_desaturation_gain/2(scale)
  inputs/1 -> compute_desaturation_gain/1(inputs)
  compute_desaturation_gain/3(k) -> [k1]
  reduce_only/1 -> Data Type Conversion/1
  [k1] -> Compare To Zero/1
  Data Type Conversion/1 -> Logical Operator/1
  Compare To Zero/1 -> Logical Operator/2
  Logical Operator/1 -> If/1
  Merge/1 -> out/1
  compute_desaturation_gain/2(motor_pos) -> [motor_pos]
  compute_desaturation_gain/1(motor_neg) -> [motor_neg]
  If/1 -> If Action Subsystem/Action
  scale1/1 -> Subsystem/2(scale)
  inputs2/1 -> Subsystem/3(inputs)
  If/2 -> Subsystem/Action
  [k1] -> Subsystem/1(k1)
  If Action Subsystem/1(out) -> Merge/1
  Subsystem/1(out) -> Merge/2
  [motor_pos] -> If Action Subsystem/2(motor_pos)
  [motor_neg] -> If Action Subsystem/1(motor_neg)
  inputs1/1 -> If Action Subsystem/3(outputs)
  min_out/1 -> compute_desaturation_gain/3(min)
  max_out/1 -> compute_desaturation_gain/4(max)

== system mixer_old/MultirotorMixer/mix_airmode_rp/mix_without_yaw ==
  four_input : Inport
  scale : Inport  Port=2
  Gain2 : Gain  Gain=[1, 1, 0, 1]
      settings: AttributesFormatString=%<Gain>
  Mux2 : Mux
  Product2 : Product
  Reshape1 : Reshape  OutputDimensionality=Customize  OutputDimensions=[4,4]
      settings: AttributesFormatString=%<OutputDimensions>
  Sum of Elements1 : Sum  Inputs=+  CollapseMode=Specified dimension  CollapseDim=2
      settings: AttributesFormatString=%<CollapseDim>
  Transpose1 : Math  Operator=transpose
  outputs : Outport
  wires:
  four_input/1 -> Gain2/1
  Gain2/1 -> Mux2/4, Mux2/3, Mux2/2, Mux2/1
  Mux2/1 -> Reshape1/1
  Reshape1/1 -> Transpose1/1
  scale/1 -> Product2/2
  Product2/1 -> Sum of Elements1/1
  Sum of Elements1/1 -> outputs/1
  Transpose1/1 -> Product2/1

== system mixer_old/MultirotorMixer/mix_airmode_rp/mix_yaw ==
  inputs : Inport
  four_input : Inport  Port=2
  scale : Inport  Port=3
  Bus Selector1 : BusSelector  OutputSignals=outputs
  Bus Selector2 : BusSelector  OutputSignals=outputs
  Constant : Constant  Value=0  OutDataTypeStr=single
  Constant1 : Constant  Value=1.15  OutDataTypeStr=single
  Constant2 : Constant  Value=0  OutDataTypeStr=single
  Constant3 : Constant  Value=0  OutDataTypeStr=single
  Constant4 : Constant  OutDataTypeStr=single
  Constant5 : Constant  OutDataTypeStr=single
  Product : Product
  Selector : Selector  InputPortWidth=4  IndexOptions=Index vector (dialog)  Indices=3  OutputSizes=1
  Selector1 : Selector  NumberOfDimensions=2  InputPortWidth=3  IndexOptions=Select all,Index vector (dialog)  Indices=[1 3],3  OutputSizes=1,1
  Sum : Sum  Inputs=++|
  minimize_saturation2 : Subsystem
  minimize_saturation3 : Subsystem
  scale1 : InportShadow  Port=3
  scale2 : InportShadow  Port=3
  out : Outport
  wires:
  four_input/1 -> Selector/1
  Selector/1 -> Product/1  "yaw"
  Product/1 -> Sum/2
  inputs/1 -> Bus Selector1/1
  scale/1 -> Selector1/1
  Selector1/1 -> Product/2  "yaw_scale"
  Bus Selector1/1 -> Sum/1  "<outputs>"
  Sum/1 -> minimize_saturation2/1(inputs)  "outputs"
  scale1/1 -> minimize_saturation2/2(scale)
  Constant2/1 -> minimize_saturation2/5(reduce_only)
  Constant1/1 -> minimize_saturation2/4(max_out)
  Constant/1 -> minimize_saturation2/3(min_out)
  minimize_saturation2/1(out) -> Bus Selector2/1
  Bus Selector2/1 -> minimize_saturation3/1(inputs)  "<outputs>"
  scale2/1 -> minimize_saturation3/2(scale)
  Constant5/1 -> minimize_saturation3/5(reduce_only)
  Constant3/1 -> minimize_saturation3/3(min_out)
  Constant4/1 -> minimize_saturation3/4(max_out)
  minimize_saturation3/1(out) -> out/1

== system mixer_old/MultirotorMixer/mix_airmode_rpy/full_mixing ==
  four_input : Inport
  scale : Inport  Port=2
  Mux2 : Mux
  Product2 : Product
  Reshape1 : Reshape  OutputDimensionality=Customize  OutputDimensions=[4,4]
      settings: AttributesFormatString=%<OutputDimensions>
  Sum of Elements1 : Sum  Inputs=+  CollapseMode=Specified dimension  CollapseDim=2
      settings: AttributesFormatString=%<CollapseDim>
  Transpose1 : Math  Operator=transpose
  outputs : Outport
  wires:
  four_input/1 -> Mux2/4, Mux2/3, Mux2/2, Mux2/1
  Mux2/1 -> Reshape1/1
  Reshape1/1 -> Transpose1/1
  scale/1 -> Product2/2
  Product2/1 -> Sum of Elements1/1
  Sum of Elements1/1 -> outputs/1
  Transpose1/1 -> Product2/1

== system mixer_old/MultirotorMixer/mix_airmode_rpy/minimize_saturation ==
  inputs : Inport
  scale : Inport  Port=2
  min_out : Inport  Port=3
  max_out : Inport  Port=4
  reduce_only : Inport  Port=5
  Compare To Zero : simulink/Logic and Bit Operations/Compare To Zero  relop=>  OutDataTypeStr=boolean
  Data Type Conversion : DataTypeConversion  OutDataTypeStr=boolean  SaturateOnIntegerOverflow=off  RndMeth=Floor
  If : If  IfExpression=u1
  If Action Subsystem : Subsystem  TreatAsAtomicUnit=on
  Logical Operator : Logic  AllPortsSameDT=off  OutDataTypeStr=boolean
  Merge : Merge
  Subsystem : Subsystem
  compute_desaturation_gain : Subsystem
  inputs1 : InportShadow
  inputs2 : InportShadow
  scale1 : InportShadow  Port=2
  out : Outport
  wires:
  scale/1 -> compute_desaturation_gain/2(scale)
  inputs/1 -> compute_desaturation_gain/1(inputs)
  compute_desaturation_gain/3(k) -> [k1]
  reduce_only/1 -> Data Type Conversion/1
  [k1] -> Compare To Zero/1
  Data Type Conversion/1 -> Logical Operator/1
  Compare To Zero/1 -> Logical Operator/2
  Logical Operator/1 -> If/1
  Merge/1 -> out/1
  compute_desaturation_gain/2(motor_pos) -> [motor_pos]
  compute_desaturation_gain/1(motor_neg) -> [motor_neg]
  If/1 -> If Action Subsystem/Action
  scale1/1 -> Subsystem/2(scale)
  inputs2/1 -> Subsystem/3(inputs)
  If/2 -> Subsystem/Action
  [k1] -> Subsystem/1(k1)
  If Action Subsystem/1(out) -> Merge/1
  Subsystem/1(out) -> Merge/2
  [motor_pos] -> If Action Subsystem/2(motor_pos)
  [motor_neg] -> If Action Subsystem/1(motor_neg)
  inputs1/1 -> If Action Subsystem/3(outputs)
  min_out/1 -> compute_desaturation_gain/3(min)
  max_out/1 -> compute_desaturation_gain/4(max)

== system mixer_old/MultirotorMixer/mix_airmode_rpy/minimize_saturation1 ==
  inputs : Inport
  scale : Inport  Port=2
  min_out : Inport  Port=3
  max_out : Inport  Port=4
  reduce_only : Inport  Port=5
  Compare To Zero : simulink/Logic and Bit Operations/Compare To Zero  relop=>  OutDataTypeStr=boolean
  Data Type Conversion : DataTypeConversion  OutDataTypeStr=boolean  SaturateOnIntegerOverflow=off  RndMeth=Floor
  If : If  IfExpression=u1
  If Action Subsystem : Subsystem  TreatAsAtomicUnit=on
  Logical Operator : Logic  AllPortsSameDT=off  OutDataTypeStr=boolean
  Merge : Merge
  Subsystem : Subsystem
  compute_desaturation_gain : Subsystem
  inputs1 : InportShadow
  inputs2 : InportShadow
  scale1 : InportShadow  Port=2
  out : Outport
  wires:
  max_out/1 -> compute_desaturation_gain/4(max)
  min_out/1 -> compute_desaturation_gain/3(min)
  inputs1/1 -> If Action Subsystem/3(outputs)
  [motor_neg] -> If Action Subsystem/1(motor_neg)
  [motor_pos] -> If Action Subsystem/2(motor_pos)
  Subsystem/1(out) -> Merge/2
  If Action Subsystem/1(out) -> Merge/1
  [k1] -> Subsystem/1(k1)
  If/2 -> Subsystem/Action
  inputs2/1 -> Subsystem/3(inputs)
  scale1/1 -> Subsystem/2(scale)
  If/1 -> If Action Subsystem/Action
  compute_desaturation_gain/1(motor_neg) -> [motor_neg]
  compute_desaturation_gain/2(motor_pos) -> [motor_pos]
  Merge/1 -> out/1
  Logical Operator/1 -> If/1
  Compare To Zero/1 -> Logical Operator/2
  Data Type Conversion/1 -> Logical Operator/1
  [k1] -> Compare To Zero/1
  reduce_only/1 -> Data Type Conversion/1
  compute_desaturation_gain/3(k) -> [k1]
  inputs/1 -> compute_desaturation_gain/1(inputs)
  scale/1 -> compute_desaturation_gain/2(scale)

== system mixer_old/MultirotorMixer/apply_thrust_model/slew_rate_limit/cal_delta_out_max ==
  MOT_SLEW_MAX : Inport
  Compare To Constant : simulink/Logic and Bit Operations/Compare To Constant  relop=>  const=eps  OutDataTypeStr=boolean
  Constant1 : Constant  Value=0  OutDataTypeStr=single
  Data Type Conversion : DataTypeConversion  OutDataTypeStr=uint8  SaturateOnIntegerOverflow=off  RndMeth=Floor
  If Action Subsystem : Subsystem  TreatAsAtomicUnit=on
  If Action Subsystem1 : Subsystem  TreatAsAtomicUnit=on
  MOT_SLEW_MAX1 : InportShadow
  Merge : Merge
  Switch Case : SwitchCase
  delta_out_max : Outport
  wires:
  MOT_SLEW_MAX/1 -> Compare To Constant/1
  Switch Case/1 -> If Action Subsystem/Action
  Switch Case/2 -> If Action Subsystem1/Action
  Merge/1 -> delta_out_max/1
  If Action Subsystem/1(Out1) -> Merge/1
  If Action Subsystem1/1(Out1) -> Merge/2
  Constant1/1 -> If Action Subsystem1/1(In1)
  MOT_SLEW_MAX1/1 -> If Action Subsystem/1(MOT_SLEW_MAX)
  Compare To Constant/1 -> Data Type Conversion/1
  Data Type Conversion/1 -> Switch Case/1

== system mixer_old/MultirotorMixer/mix_airmode_disabled/minimize_saturation/If Action Subsystem ==
  motor_neg : Inport
  motor_pos : Inport  Port=2
  outputs : Inport  Port=3
  Action Port : ActionPort  ActionPortLabel=if(u1)
  Bus Creator : BusCreator  Inputs=3
  out : Outport
  wires:
  motor_pos/1 -> Bus Creator/2  "motor_pos"
  motor_neg/1 -> Bus Creator/1  "motor_neg"
  outputs/1 -> Bus Creator/3  "outputs"
  Bus Creator/1 -> out/1

== system mixer_old/MultirotorMixer/mix_airmode_disabled/minimize_saturation/Subsystem ==
  k1 : Inport
  scale : Inport  Port=2
  inputs : Inport  Port=3
  Action Port : ActionPort  ActionPortLabel=else
  Bus Creator1 : BusCreator  Inputs=3
  Constant1 : Constant  Value=0  OutDataTypeStr=single
  Constant2 : Constant  OutDataTypeStr=single
  Gain : Gain  Gain=0.5
  Product : Product
  Product1 : Product
  Selector : Selector  NumberOfDimensions=2  InputPortWidth=3  IndexOptions=Select all,Index vector (dialog)  Indices=[1 3],4  OutputSizes=1,1
  Selector1 : Selector  NumberOfDimensions=2  InputPortWidth=3  IndexOptions=Select all,Index vector (dialog)  Indices=[1 3],4  OutputSizes=1,1
  Sum : Sum  Inputs=++|
  Sum1 : Sum  Inputs=|++
  compute_desaturation_gain : Subsystem
  scale1 : InportShadow  Port=2
  scale2 : InportShadow  Port=2
  out : Outport
  wires:
  Sum/1 -> compute_desaturation_gain/1(inputs), Sum1/2
  scale/1 -> Selector/1
  compute_desaturation_gain/2(motor_pos) -> Bus Creator1/2  "motor_pos"
  Sum1/1 -> Bus Creator1/3  "outputs"
  compute_desaturation_gain/3(k) -> Gain/1
  Product1/1 -> Sum1/1
  compute_desaturation_gain/1(motor_neg) -> Bus Creator1/1  "motor_neg"
  Bus Creator1/1 -> out/1
  Gain/1 -> Product1/1  "k2"
  k1/1 -> Product/1
  Constant1/1 -> compute_desaturation_gain/3(min)
  Constant2/1 -> compute_desaturation_gain/4(max)
  Selector/1 -> Product/2  "desat"
  Product/1 -> Sum/2
  inputs/1 -> Sum/1
  scale1/1 -> compute_desaturation_gain/2(scale)
  scale2/1 -> Selector1/1
  Selector1/1 -> Product1/2  "desat"
